simulink library "inp"  (R2021b)
settings: Solver=VariableStepAuto  StartTime=0.0  StopTime=10.0  RelTol=1e-3
undefined symbols (not defined in the file): C_TASK_5MS_S, FALSE, KINP_AcoreReadyToSlp_flg_ovrdflg, KINP_AcoreReadyToSlp_flg_ovrdval, KINP_AllowMovThd_OTA_enum_ovrdflg, KINP_AllowMovThd_OTA_enum_ovrdval, KINP_APSAngleTarget_Deg_ovrdflg, KINP_APSAngleTarget_Deg_ovrdval, KINP_APSDecReq_mps2_ovrdflg, KINP_APSDecReq_mps2_ovrdval, KINP_APSDecReqA_flg_ovrdflg, KINP_APSDecReqA_flg_ovrdval, KINP_APSDFLL_cm_ovrdflg, KINP_APSDFLL_cm_ovrdval, KINP_APSDFLR_cm_ovrdflg, KINP_APSDFLR_cm_ovrdval, KINP_APSDRLL_cm_ovrdflg, KINP_APSDRLL_cm_ovrdval, KINP_APSDRLR_cm_ovrdflg, KINP_APSDRLR_cm_ovrdval, KINP_APSExitCondition_enum_ovrdflg, KINP_APSExitCondition_enum_ovrdval, KINP_APSHWVer_enum_ovrdflg, KINP_APSHWVer_enum_ovrdval, KINP_APSProgressPCT_pct_ovrdflg, KINP_APSProgressPCT_pct_ovrdval, KINP_APSReq_enum_ovrdflg, KINP_APSReq_enum_ovrdval, KINP_APSRQDisplay_enum_ovrdflg, KINP_APSRQDisplay_enum_ovrdval, KINP_APSRqEPASCtrl_flg_ovrdflg, KINP_APSRqEPASCtrl_flg_ovrdval, KINP_APSShiftPosnReq_enum_ovrdval, KINP_APSShiftPosnReq_enum_ovrflg, KINP_APSSpeedCMD_kph_ovrdval, KINP_APSSpeedCMD_kph_ovrflg, KINP_APSStaSystem_enum_ovrdflg, KINP_APSStaSystem_enum_ovrdval, KINP_APSSWVer_enum_ovrdflg, KINP_APSSWVer_enum_ovrdval, KINP_APSVMCReqA_flg_ovrdval, KINP_APSVMCReqA_flg_ovrflg, KINP_APSVRqEPASCtrl_flg_ovrdflg, KINP_APSVRqEPASCtrl_flg_ovrdval, KINP_AuxBattVolmV_mV_ovrdflg, KINP_AuxBattVolmV_mV_ovrdval, KINP_CAASSta_enum_ovrdflg, KINP_CAASSta_enum_ovrdval, KINP_CAASVMCReqA_flg_ovrdval, KINP_CAASVMCReqA_flg_ovrflg, KINP_Chime_enum_ovrdflg, KINP_Chime_enum_ovrdval, KINP_ClearDTCcmd_flg_ovrdflg, KINP_ClearDTCcmd_flg_ovrdval, KINP_EvccAplusPwrUpReq_flg_ovrdflg, KINP_EvccAplusPwrUpReq_flg_ovrdval, KINP_LFID_raw_ovrdval, KINP_LFID_raw_ovrflg, KINP_LRID_raw_ovrdval, KINP_MemOffsetAccX_raw16_ovrdflg ... (+118)
libraries: FVT_lib x942, hcu_lib x1
(part 2 of 31)

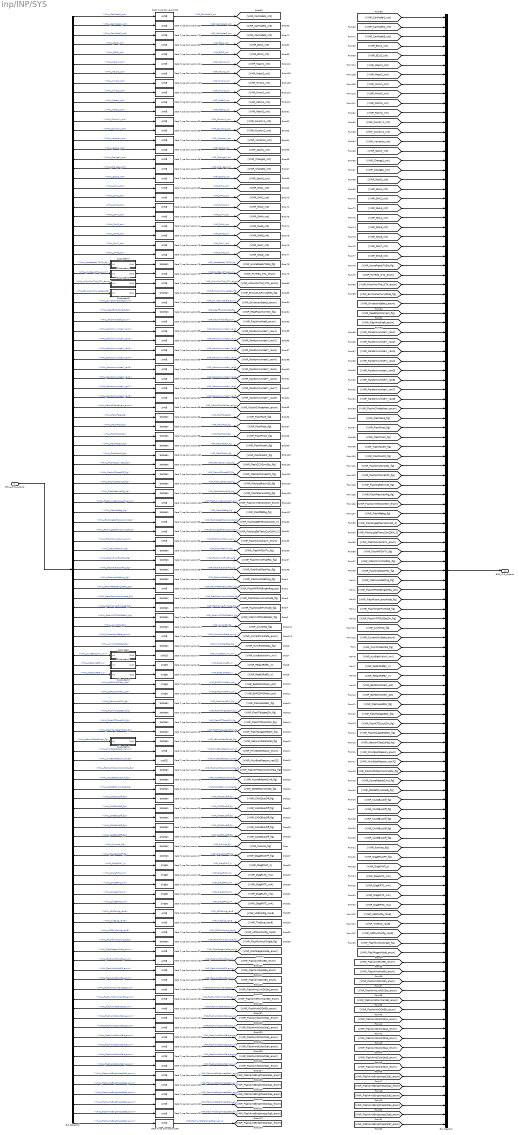
== system inp/INP/SYS ==
  BHAL_SYS_outputs : Inport  OutDataTypeStr=Bus: BHAL_SYS_outputs
  Bus Creator1 : BusCreator  Inputs=117
  Bus Selector1 : BusSelector  OutputSignals=VHAL_CarMode1_cnt,VHAL_CarModel2_cnt,VHAL_CarModel3_cnt,VHAL_ECU1_cnt,VHAL_ECU2_cnt,VHAL_Major1_cnt,VHAL_Major2_cnt,VHAL_Minor1_cnt,VHAL_Minor2_cnt,VHAL_Patch1_cnt,VHAL_Patch2_cnt,VHAL_Country1_cnt,VHAL_Country2_cnt,VHAL_Variation_cnt,VHAL_Dash1_cnt,VHAL_Change1_cnt,VHAL_Change2_cnt,VHAL_Dash2_cnt,VHAL_SHA1_cnt,VHAL_SHA2_cnt,VHAL_SHA3_cnt,VHAL_SHA4_cnt,VHAL_SHA5_cnt,VHAL_SHA6_cnt,VHAL_SHA7_cnt,VHAL_SHA8_cnt,VHAL_AcoreReadyToSlp_flg,VHAL_PwrReq_OTA_enum,VHAL_AllowMovThd_OTA_enum,VHAL_EvccAplusPwrUpReq_flg,VHAL_DrivetrainSelect_enum,VHAL_ReadFlashCorrect_flg,VHAL_FlashAntitheft_enum,VHAL_RandomnumberY_raw1,VHAL_RandomnumberY_raw2,VHAL_RandomnumberY_raw3,VHAL_RandomnumberY_raw4,VHAL_RandomnumberY_raw5,VHAL_RandomnumberY_raw6,VHAL_RandomnumberY_raw7,VHAL_RandomnumberY_raw8,VHAL_FlashACModeMem_enum,VHAL_FlashFace_flg,VHAL_FlashFoot_flg,VHAL_FlashFrost_flg,VHAL_FlashFaceM_flg,VHAL_FlashFootM_flg,VHAL_FlashCCUSyncSts_flg,VHAL_FlashACForceOFF_flg,VHAL_FlashsigRecircSt_flg,VHAL_FlashRecAutoFlg_flg,VHAL_FlashAirIntenZone1M_enum,VHAL_Flashfdefog_flg,VHAL_FlashsigSetTempZon1St_C,VHAL_FlashsigSetTempZon2StM_C,VHAL_FlashCountAlarm_enum,VHAL_FlashMFSWTri_flg,VHAL_FlashMirrorFlodPos_flg,VHAL_FlashFuelDoorPos_flg,VHAL_FlashLockSetting_flg,VHAL_FlashMFRDNBrightReq_pct,VHAL_FlashRoomLampMode_flg,VHAL_FlashWiperFixMode_flg,VHAL_FlashIVIPTGUSStaSW_flg,VHAL_AnyNMID_flg,VHAL_CurrentNmState_enum,VHAL_NvmProtectSta_flg,VHAL_AuxBattVolmV_mV,VHAL_Pedal1Ref5V_V,VHAL_Pedal2Ref5V_V,VHAL_EAPS1MINMem_pct,VHAL_EAPS2MINMem_pct,VHAL_FlashHoodSW_flg,VHAL_FlashTailgateSW_flg,VHAL_FlashCTDLockSW_flg,VHAL_FlashTailgateHDSW_flg,VHAL_NetworkReqCalled_flg,VHAL_PmicBootReason_enum,VHAL_WisrBootReason_raw32,VHAL_FlashAPMDoorControlSta_flg,VHAL_AcoreRebootCmd_flg,VHAL_DIDGetDynoMode_flg,VHAL_CAN1BusOff_flg,VHAL_CAN2BusOff_flg,VHAL_CAN3BusOff_flg,VHAL_CAN4BusOff_flg,VHAL_CAN5BusOff_flg,VHAL_funAuto_flg,VHAL_DiagDRLOFF_flg,VHAL_DiagFMHT_s,VHAL_DiagFLTC_mA,VHAL_DiagFRTC_mA,VHAL_DiagRLTC_mA,VHAL_DiagRRTC_mA,VHAL_USSConfig_raw8,VHAL_TireSize_raw8,VHAL_APSFunConfig_raw8,VHAL_FlashfUnlockSingle_flg,VHAL_FlashRegenMode_enum,VHAL_FlashAmbFunEN_enum,VHAL_FlashAmbWelEN_enum,VHAL_FlashAmbDimEN_enum,VHAL_FlashAmbLinkDriSta_enum,VHAL_FlashAmbPwrWarnEN_enum,VHAL_FlashAmbODAEN_enum,VHAL_FlashAmbColorSta1_enum,VHAL_FlashAmbColorSta2_enum,VHAL_FlashAmbColorSta3_enum,VHAL_FlashAmbColorSta4_enum,VHAL_FlashAmbColorSta5_enum,VHAL_FlashAmbColorSta7_enum,VHAL_FlashAmbBrightnessSta1_enum,VHAL_FlashAmbBrightnessSta2_enum,VHAL_FlashAmbBrightnessSta3_enum,VHAL_FlashAmbBrightnessSta4_enum,VHAL_FlashAmbBrightnessSta5_enum,VHAL_FlashAmbBrightnessSta7_enum
  Data Type Conversion{,1,3..6,12..16,19..27,36,54,57..58,78,81,89,96..103,105,107,112} (38 alike) : DataTypeConversion  OutDataTypeStr=boolean
  Data Type Conversion{8..11,28..32} (9 alike) : DataTypeConversion  OutDataTypeStr=single
  Data Type Conversion{2,17,33..35,37,53,55..56,59..77,79..80,82..88,90..95,104,106,108..111,113,192..209} (68 alike) : DataTypeConversion  OutDataTypeStr=uint8
  Data Type Conversion18 : DataTypeConversion  OutDataTypeStr=uint32
  Data Type Conversion7 : DataTypeConversion  OutDataTypeStr=uint16
  Subsystem : Subsystem
  Subsystem1 : Subsystem
  Subsystem2 : Subsystem
  Subsystem3 : Subsystem
  Subsystem4 : Subsystem
  Subsystem5 : Subsystem
  Subsystem6 : Subsystem
  Subsystem7 : Subsystem
  BINP_SYS_outputs : Outport  OutDataTypeStr=Bus: BINP_SYS_outputs
  wires:
  [VINP_Country2_cnt] -> Bus Creator1/13
  [VINP_FlashAirIntenZone1M_enum] -> Bus Creator1/52
  [VINP_FlashFrost_flg] -> Bus Creator1/45
  Bus Selector1/43 -> Data Type Conversion96/1  "<VHAL_FlashFace_flg>"
  [VINP_FlashCCUSyncSts_flg] -> Bus Creator1/48
  [VINP_EvccAplusPwrUpReq_flg] -> Bus Creator1/30
  Data Type Conversion110/1 -> [VINP_Minor2_cnt]  "VINP_Minor2_cnt"
  Bus Selector1/53 -> Data Type Conversion107/1  "<VHAL_Flashfdefog_flg>"
  [VINP_FlashRecAutoFlg_flg] -> Bus Creator1/51
  Bus Selector1/16 -> Data Type Conversion66/1  "<VHAL_Change1_cnt>"
  [VINP_RandomnumberY_raw1] -> Bus Creator1/34
  Data Type Conversion97/1 -> [VINP_FlashFoot_flg]  "VINP_FlashFoot_flg"
  Bus Selector1/44 -> Data Type Conversion97/1  "<VHAL_FlashFoot_flg>"
  [VINP_FlashFoot_flg] -> Bus Creator1/44
  [VINP_FlashFootM_flg] -> Bus Creator1/47
  Data Type Conversion72/1 -> [VINP_SHA3_cnt]  "VINP_SHA3_cnt"
  [VINP_FlashsigRecircSt_flg] -> Bus Creator1/50
  Data Type Conversion60/1 -> [VINP_CarModel2_cnt]  "VINP_CarModel2_cnt"
  Data Type Conversion100/1 -> [VINP_FlashFootM_flg]  "VINP_FlashFootM_flg"
  Bus Selector1/3 -> Data Type Conversion71/1  "<VHAL_CarModel3_cnt>"
  Data Type Conversion104/1 -> [VINP_Major1_cnt]  "VINP_Major1_cnt"
  [VINP_FlashFaceM_flg] -> Bus Creator1/46
  [VINP_Dash1_cnt] -> Bus Creator1/15
  Bus Selector1/45 -> Data Type Conversion98/1  "<VHAL_FlashFrost_flg>"
  [VINP_FlashACModeMem_enum] -> Bus Creator1/42
  Data Type Conversion108/1 -> [VINP_Major2_cnt]  "VINP_Major2_cnt"
  [VINP_FlashFace_flg] -> Bus Creator1/43
  Bus Selector1/8 -> Data Type Conversion109/1  "<VHAL_Minor1_cnt>"
  [VINP_CarModel1_cnt] -> Bus Creator1/1
  Data Type Conversion82/1 -> [VINP_ECU1_cnt]  "VINP_ECU1_cnt"
  Bus Selector1/47 -> Data Type Conversion100/1  "<VHAL_FlashFootM_flg>"
  Data Type Conversion73/1 -> [VINP_SHA4_cnt]  "VINP_SHA4_cnt"
  Bus Selector1/34 -> Data Type Conversion85/1  "<VHAL_RandomnumberY_raw1>"
  Data Type Conversion84/1 -> [VINP_DrivetrainSelect_enum]  "VINP_DrivetrainSelect_enum"
  Bus Selector1/30 -> Subsystem6/1(In1)  "<VHAL_EvccAplusPwrUpReq_flg>"
  Data Type Conversion101/1 -> [VINP_FlashCCUSyncSts_flg]  "VINP_FlashCCUSyncSts_flg"
  [VINP_DrivetrainSelect_enum] -> Bus Creator1/31
  Data Type Conversion80/1 -> [VINP_AllowMovThd_OTA_enum]  "VINP_AllowMovThd_OTA_enum"
  Bus Selector1/49 -> Data Type Conversion102/1  "<VHAL_FlashACForceOFF_flg>"
  Bus Selector1/38 -> Data Type Conversion90/1  "<VHAL_RandomnumberY_raw5>"
  Bus Selector1/10 -> Data Type Conversion111/1  "<VHAL_Patch1_cnt>"
  Data Type Conversion88/1 -> [VINP_RandomnumberY_raw4]  "VINP_RandomnumberY_raw4"
  [VINP_Flashfdefog_flg] -> Bus Creator1/53
  Bus Selector1/42 -> Data Type Conversion95/1  "<VHAL_FlashACModeMem_enum>"
  Bus Selector1/37 -> Data Type Conversion88/1  "<VHAL_RandomnumberY_raw4>"
  Bus Selector1/36 -> Data Type Conversion87/1  "<VHAL_RandomnumberY_raw3>"
  Bus Selector1/48 -> Data Type Conversion101/1  "<VHAL_FlashCCUSyncSts_flg>"
  Data Type Conversion102/1 -> [VINP_FlashACForceOFF_flg]  "VINP_FlashACForceOFF_flg"
  [VINP_Change2_cnt] -> Bus Creator1/17
  Bus Selector1/29 -> Subsystem5/1(In1)  "<VHAL_AllowMovThd_OTA_enum>"
  Data Type Conversion63/1 -> [VINP_Country2_cnt]  "VINP_Country2_cnt"
  Data Type Conversion107/1 -> [VINP_Flashfdefog_flg]  "VINP_Flashfdefog_flg"
  Data Type Conversion96/1 -> [VINP_FlashFace_flg]  "VINP_FlashFace_flg"
  [VINP_RandomnumberY_raw2] -> Bus Creator1/35
  [VINP_RandomnumberY_raw6] -> Bus Creator1/39
  [VINP_RandomnumberY_raw4] -> Bus Creator1/37
  [VINP_ECU1_cnt] -> Bus Creator1/4
  Bus Selector1/2 -> Data Type Conversion60/1  "<VHAL_CarModel2_cnt>"
  Data Type Conversion105/1 -> [VINP_FlashRecAutoFlg_flg]  "VINP_FlashRecAutoFlg_flg"
  Data Type Conversion103/1 -> [VINP_FlashsigRecircSt_flg]  "VINP_FlashsigRecircSt_flg"
  Bus Selector1/22 -> Data Type Conversion73/1  "<VHAL_SHA4_cnt>"
  Bus Selector1/46 -> Data Type Conversion99/1  "<VHAL_FlashFaceM_flg>"
  Bus Selector1/50 -> Data Type Conversion103/1  "<VHAL_FlashsigRecircSt_flg>"
  Data Type Conversion98/1 -> [VINP_FlashFrost_flg]  "VINP_FlashFrost_flg"
  [VINP_RandomnumberY_raw5] -> Bus Creator1/38
  [VINP_SHA3_cnt] -> Bus Creator1/21
  Bus Selector1/40 -> Data Type Conversion92/1  "<VHAL_RandomnumberY_raw7>"
  Data Type Conversion86/1 -> [VINP_RandomnumberY_raw2]  "VINP_RandomnumberY_raw2"
  Data Type Conversion111/1 -> [VINP_Patch1_cnt]  "VINP_Patch1_cnt"
  Bus Selector1/35 -> Data Type Conversion86/1  "<VHAL_RandomnumberY_raw2>"
  [VINP_SHA6_cnt] -> Bus Creator1/24
  [VINP_Major1_cnt] -> Bus Creator1/6
  [VINP_RandomnumberY_raw7] -> Bus Creator1/40
  [VINP_RandomnumberY_raw8] -> Bus Creator1/41
  Bus Selector1/15 -> Data Type Conversion65/1  "<VHAL_Dash1_cnt>"
  Data Type Conversion92/1 -> [VINP_RandomnumberY_raw7]  "VINP_RandomnumberY_raw7"
  Data Type Conversion99/1 -> [VINP_FlashFaceM_flg]  "VINP_FlashFaceM_flg"
  Data Type Conversion85/1 -> [VINP_RandomnumberY_raw1]  "VINP_RandomnumberY_raw1"
  Bus Selector1/52 -> Data Type Conversion106/1  "<VHAL_FlashAirIntenZone1M_enum>"
  Data Type Conversion90/1 -> [VINP_RandomnumberY_raw5]  "VINP_RandomnumberY_raw5"
  Data Type Conversion91/1 -> [VINP_RandomnumberY_raw6]  "VINP_RandomnumberY_raw6"
  Data Type Conversion65/1 -> [VINP_Dash1_cnt]  "VINP_Dash1_cnt"
  [VINP_FlashAntitheft_enum] -> Bus Creator1/33
  Data Type Conversion87/1 -> [VINP_RandomnumberY_raw3]  "VINP_RandomnumberY_raw3"
  Bus Selector1/39 -> Data Type Conversion91/1  "<VHAL_RandomnumberY_raw6>"
  [VINP_Dash2_cnt] -> Bus Creator1/18
  Bus Selector1/19 -> Data Type Conversion69/1  "<VHAL_SHA1_cnt>"
  Bus Selector1/41 -> Data Type Conversion94/1  "<VHAL_RandomnumberY_raw8>"
  Data Type Conversion71/1 -> [VINP_CarModel3_cnt]  "VINP_CarModel3_cnt"
  [VINP_SHA4_cnt] -> Bus Creator1/22
  Data Type Conversion76/1 -> [VINP_SHA7_cnt]  "VINP_SHA7_cnt"
  [VINP_AllowMovThd_OTA_enum] -> Bus Creator1/29
  [VINP_ReadFlashCorrect_flg] -> Bus Creator1/32
  Data Type Conversion78/1 -> [VINP_AcoreReadyToSlp_flg]  "VINP_AcoreReadyToSlp_flg"
  Data Type Conversion94/1 -> [VINP_RandomnumberY_raw8]  "VINP_RandomnumberY_raw8"
  Data Type Conversion67/1 -> [VINP_Change2_cnt]  "VINP_Change2_cnt"
  [VINP_CarModel3_cnt] -> Bus Creator1/3
  [VINP_Variation_cnt] -> Bus Creator1/14
  [VINP_SHA2_cnt] -> Bus Creator1/20
  [VINP_FlashACForceOFF_flg] -> Bus Creator1/49
  Bus Selector1/12 -> Data Type Conversion62/1  "<VHAL_Country1_cnt>"
  Bus Selector1/51 -> Data Type Conversion105/1  "<VHAL_FlashRecAutoFlg_flg>"
  Data Type Conversion69/1 -> [VINP_SHA1_cnt]  "VINP_SHA1_cnt"
  [VINP_AcoreReadyToSlp_flg] -> Bus Creator1/27
  [VINP_PwrReq_OTA_enum] -> Bus Creator1/28
  Subsystem4/1(Out1) -> Data Type Conversion79/1
  [VINP_SHA5_cnt] -> Bus Creator1/23
  [VINP_Patch2_cnt] -> Bus Creator1/11
  [VINP_Patch1_cnt] -> Bus Creator1/10
  Data Type Conversion68/1 -> [VINP_Dash2_cnt]  "VINP_Dash2_cnt"
  Subsystem6/1(Out1) -> Data Type Conversion89/1
  Bus Selector1/33 -> Data Type Conversion83/1  "<VHAL_FlashAntitheft_enum>"
  [VINP_Minor2_cnt] -> Bus Creator1/9
  [VINP_SHA7_cnt] -> Bus Creator1/25
  [VINP_Minor1_cnt] -> Bus Creator1/8
  Data Type Conversion95/1 -> [VINP_FlashACModeMem_enum]  "VINP_FlashACModeMem_enum"
  [VINP_CarModel2_cnt] -> Bus Creator1/2
  Data Type Conversion77/1 -> [VINP_SHA8_cnt]  "VINP_SHA8_cnt"
  Data Type Conversion106/1 -> [VINP_FlashAirIntenZone1M_enum]  "VINP_FlashAirIntenZone1M_enum"
  Data Type Conversion66/1 -> [VINP_Change1_cnt]  "VINP_Change1_cnt"
  [VINP_SHA1_cnt] -> Bus Creator1/19
  Data Type Conversion81/1 -> [VINP_ReadFlashCorrect_flg]  "VINP_ReadFlashCorrect_flg"
  [VINP_Country1_cnt] -> Bus Creator1/12
  Bus Selector1/17 -> Data Type Conversion67/1  "<VHAL_Change2_cnt>"
  Data Type Conversion83/1 -> [VINP_FlashAntitheft_enum]  "VINP_FlashAntitheft_enum"
  Data Type Conversion75/1 -> [VINP_SHA6_cnt]  "VINP_SHA6_cnt"
  Data Type Conversion74/1 -> [VINP_SHA5_cnt]  "VINP_SHA5_cnt"
  Data Type Conversion93/1 -> [VINP_ECU2_cnt]  "VINP_ECU2_cnt"
  [VINP_RandomnumberY_raw3] -> Bus Creator1/36
  Data Type Conversion70/1 -> [VINP_SHA2_cnt]  "VINP_SHA2_cnt"
  Bus Selector1/21 -> Data Type Conversion72/1  "<VHAL_SHA3_cnt>"
  Data Type Conversion62/1 -> [VINP_Country1_cnt]  "VINP_Country1_cnt"
  [VINP_ECU2_cnt] -> Bus Creator1/5
  Bus Selector1/31 -> Data Type Conversion84/1  "<VHAL_DrivetrainSelect_enum>"
  Data Type Conversion64/1 -> [VINP_Variation_cnt]  "VINP_Variation_cnt"
  Data Type Conversion61/1 -> [VINP_Patch2_cnt]  "VINP_Patch2_cnt"
  Bus Selector1/18 -> Data Type Conversion68/1  "<VHAL_Dash2_cnt>"
  Bus Selector1/28 -> Subsystem4/1(In1)  "<VHAL_PwrReq_OTA_enum>"
  Bus Selector1/24 -> Data Type Conversion75/1  "<VHAL_SHA6_cnt>"
  Bus Selector1/27 -> Subsystem7/1(In1)  "<VHAL_AcoreReadyToSlp_flg>"
  [VINP_SHA8_cnt] -> Bus Creator1/26
  Bus Selector1/20 -> Data Type Conversion70/1  "<VHAL_SHA2_cnt>"
  Subsystem5/1(Out1) -> Data Type Conversion80/1
  Bus Selector1/25 -> Data Type Conversion76/1  "<VHAL_SHA7_cnt>"
  [VINP_Major2_cnt] -> Bus Creator1/7
  Bus Selector1/32 -> Data Type Conversion81/1  "<VHAL_ReadFlashCorrect_flg>"
  Data Type Conversion59/1 -> [VINP_CarModel1_cnt]  "VINP_CarModel1_cnt"
  Bus Selector1/23 -> Data Type Conversion74/1  "<VHAL_SHA5_cnt>"
  Bus Selector1/14 -> Data Type Conversion64/1  "<VHAL_Variation_cnt>"
  [VINP_Change1_cnt] -> Bus Creator1/16
  Subsystem7/1(Out1) -> Data Type Conversion78/1
  Bus Selector1/13 -> Data Type Conversion63/1  "<VHAL_Country2_cnt>"
  Bus Selector1/4 -> Data Type Conversion82/1  "<VHAL_ECU1_cnt>"
  Data Type Conversion79/1 -> [VINP_PwrReq_OTA_enum]  "VINP_PwrReq_OTA_enum"
  Bus Selector1/7 -> Data Type Conversion108/1  "<VHAL_Major2_cnt>"
  Bus Selector1/9 -> Data Type Conversion110/1  "<VHAL_Minor2_cnt>"
  Bus Selector1/5 -> Data Type Conversion93/1  "<VHAL_ECU2_cnt>"
  Data Type Conversion89/1 -> [VINP_EvccAplusPwrUpReq_flg]  "VINP_EvccAplusPwrUpReq_flg"
  Bus Selector1/1 -> Data Type Conversion59/1  "<VHAL_CarMode1_cnt>"
  Bus Selector1/6 -> Data Type Conversion104/1  "<VHAL_Major1_cnt>"
  Data Type Conversion109/1 -> [VINP_Minor1_cnt]  "VINP_Minor1_cnt"
  BHAL_SYS_outputs/1 -> Bus Selector1/1
  Bus Creator1/1 -> BINP_SYS_outputs/1
  Bus Selector1/11 -> Data Type Conversion61/1  "<VHAL_Patch2_cnt>"
  Bus Selector1/26 -> Data Type Conversion77/1  "<VHAL_SHA8_cnt>"
  Data Type Conversion112/1 -> [VINP_AnyNMID_flg]  "VINP_AnyNMID_flg"
  Data Type Conversion113/1 -> [VINP_CurrentNmState_enum]  "VINP_CurrentNmState_enum"
  Bus Selector1/65 -> Data Type Conversion112/1  "<VHAL_AnyNMID_flg>"
  Bus Selector1/66 -> Data Type Conversion113/1  "<VHAL_CurrentNmState_enum>"
  Data Type Conversion56/1 -> [VINP_FlashCountAlarm_enum]  "VINP_FlashCountAlarm_enum"
  Data Type Conversion4/1 -> [VINP_FlashWiperFixMode_flg]  "VINP_FlashWiperFixMode_flg"
  Data Type Conversion3/1 -> [VINP_FlashRoomLampMode_flg]  "VINP_FlashRoomLampMode_flg"
  Data Type Conversion57/1 -> [VINP_FlashMirrorFlodPos_flg]  "VINP_FlashMirrorFlodPos_flg"
  Data Type Conversion55/1 -> [VINP_FlashsigSetTempZon2StM_C]  "VINP_FlashsigSetTempZon2StM_C"
  Data Type Conversion54/1 -> [VINP_FlashMFSWTri_flg]  "VINP_FlashMFSWTri_flg"
  Data Type Conversion58/1 -> [VINP_FlashFuelDoorPos_flg]  "VINP_FlashFuelDoorPos_flg"
  Data Type Conversion53/1 -> [VINP_FlashsigSetTempZon1St_C]  "VINP_FlashsigSetTempZon1St_C"
  Data Type Conversion5/1 -> [VINP_FlashIVIPTGUSStaSW_flg]  "VINP_FlashIVIPTGUSStaSW_flg"
  Data Type Conversion2/1 -> [VINP_FlashMFRDNBrightReq_pct]  "VINP_FlashMFRDNBrightReq_pct"
  Data Type Conversion1/1 -> [VINP_FlashLockSetting_flg]  "VINP_FlashLockSetting_flg"
  Bus Selector1/54 -> Data Type Conversion53/1  "<VHAL_FlashsigSetTempZon1St_C>"
  Bus Selector1/55 -> Data Type Conversion55/1  "<VHAL_FlashsigSetTempZon2StM_C>"
  Bus Selector1/56 -> Data Type Conversion56/1  "<VHAL_FlashCountAlarm_enum>"
  Bus Selector1/57 -> Data Type Conversion54/1  "<VHAL_FlashMFSWTri_flg>"
  Bus Selector1/58 -> Data Type Conversion57/1  "<VHAL_FlashMirrorFlodPos_flg>"
  Bus Selector1/59 -> Data Type Conversion58/1  "<VHAL_FlashFuelDoorPos_flg>"
  Bus Selector1/60 -> Data Type Conversion1/1  "<VHAL_FlashLockSetting_flg>"
  Bus Selector1/61 -> Data Type Conversion2/1  "<VHAL_FlashMFRDNBrightReq_pct>"
  Bus Selector1/62 -> Data Type Conversion3/1  "<VHAL_FlashRoomLampMode_flg>"
  Bus Selector1/63 -> Data Type Conversion4/1  "<VHAL_FlashWiperFixMode_flg>"
  Bus Selector1/64 -> Data Type Conversion5/1  "<VHAL_FlashIVIPTGUSStaSW_flg>"
  [VINP_FlashsigSetTempZon1St_C] -> Bus Creator1/54
  [VINP_FlashsigSetTempZon2StM_C] -> Bus Creator1/55
  [VINP_FlashCountAlarm_enum] -> Bus Creator1/56
  [VINP_FlashMFSWTri_flg] -> Bus Creator1/57
  [VINP_FlashMirrorFlodPos_flg] -> Bus Creator1/58
  [VINP_FlashFuelDoorPos_flg] -> Bus Creator1/59
  [VINP_FlashLockSetting_flg] -> Bus Creator1/60
  [VINP_FlashMFRDNBrightReq_pct] -> Bus Creator1/61
  [VINP_FlashRoomLampMode_flg] -> Bus Creator1/62
  [VINP_FlashWiperFixMode_flg] -> Bus Creator1/63
  [VINP_FlashIVIPTGUSStaSW_flg] -> Bus Creator1/64
  [VINP_AnyNMID_flg] -> Bus Creator1/65
  [VINP_CurrentNmState_enum] -> Bus Creator1/66
  Bus Selector1/67 -> Data Type Conversion6/1  "<VHAL_NvmProtectSta_flg>"
  Data Type Conversion6/1 -> [VINP_NvmProtectSta_flg]  "VINP_NvmProtectSta_flg"
  [VINP_NvmProtectSta_flg] -> Bus Creator1/67
  Bus Selector1/68 -> Subsystem/1(In1)  "<VHAL_AuxBattVolmV_mV>"
  Bus Selector1/69 -> Subsystem2/1(In1)  "<VHAL_Pedal1Ref5V_V>"
  Bus Selector1/70 -> Subsystem3/1(In1)  "<VHAL_Pedal2Ref5V_V>"
  Bus Selector1/71 -> Data Type Conversion10/1  "<VHAL_EAPS1MINMem_pct>"
  Bus Selector1/72 -> Data Type Conversion11/1  "<VHAL_EAPS2MINMem_pct>"
  Data Type Conversion7/1 -> [VINP_AuxBattVolmV_mV]  "VINP_AuxBattVolmV_mV"
  Data Type Conversion8/1 -> [VINP_Pedal1Ref5V_V]  "VINP_Pedal1Ref5V_V"
  Data Type Conversion9/1 -> [VINP_Pedal2Ref5V_V]  "VINP_Pedal2Ref5V_V"
  Data Type Conversion10/1 -> [VINP_EAPS1MINMem_pct]  "VINP_EAPS1MINMem_pct"
  Data Type Conversion11/1 -> [VINP_EAPS2MINMem_pct]  "VINP_EAPS2MINMem_pct"
  [VINP_AuxBattVolmV_mV] -> Bus Creator1/68
  [VINP_Pedal1Ref5V_V] -> Bus Creator1/69
  [VINP_Pedal2Ref5V_V] -> Bus Creator1/70
  [VINP_EAPS1MINMem_pct] -> Bus Creator1/71
  [VINP_EAPS2MINMem_pct] -> Bus Creator1/72
  Bus Selector1/73 -> Data Type Conversion12/1  "<VHAL_FlashHoodSW_flg>"
  Bus Selector1/74 -> Data Type Conversion13/1  "<VHAL_FlashTailgateSW_flg>"
  Bus Selector1/75 -> Data Type Conversion14/1  "<VHAL_FlashCTDLockSW_flg>"
  Bus Selector1/76 -> Data Type Conversion15/1  "<VHAL_FlashTailgateHDSW_flg>"
  Data Type Conversion12/1 -> [VINP_FlashHoodSW_flg]  "VINP_FlashHoodSW_flg"
  Data Type Conversion13/1 -> [VINP_FlashTailgateSW_flg]  "VINP_FlashTailgateSW_flg"
  Data Type Conversion14/1 -> [VINP_FlashCTDLockSW_flg]  "VINP_FlashCTDLockSW_flg"
  Data Type Conversion15/1 -> [VINP_FlashTailgateHDSW_flg]  "VINP_FlashTailgateHDSW_flg"
  [VINP_FlashHoodSW_flg] -> Bus Creator1/73
  [VINP_FlashTailgateSW_flg] -> Bus Creator1/74
  [VINP_FlashCTDLockSW_flg] -> Bus Creator1/75
  [VINP_FlashTailgateHDSW_flg] -> Bus Creator1/76
  Subsystem/1(Out1) -> Data Type Conversion7/1
  Bus Selector1/77 -> Subsystem1/1(In1)  "<VHAL_NetworkReqCalled_flg>"
  Data Type Conversion16/1 -> [VINP_NetworkReqCalled_flg]  "VINP_NetworkReqCalled_flg"
  Subsystem1/1(Out1) -> Data Type Conversion16/1
  [VINP_NetworkReqCalled_flg] -> Bus Creator1/77
  Bus Selector1/78 -> Data Type Conversion17/1  "<VHAL_PmicBootReason_enum>"
  Bus Selector1/79 -> Data Type Conversion18/1  "<VHAL_WisrBootReason_raw32>"
  Bus Selector1/80 -> Data Type Conversion19/1  "<VHAL_FlashAPMDoorControlSta_flg>"
  Data Type Conversion17/1 -> [VINP_PmicBootReason_enum]  "VINP_PmicBootReason_enum"
  Data Type Conversion18/1 -> [VINP_WisrBootReason_raw32]  "VINP_WisrBootReason_raw32"
  Data Type Conversion19/1 -> [VINP_FlashAPMDoorControlSta_flg]  "VINP_FlashAPMDoorControlSta_flg"
  [VINP_PmicBootReason_enum] -> Bus Creator1/78
  [VINP_WisrBootReason_raw32] -> Bus Creator1/79
  [VINP_FlashAPMDoorControlSta_flg] -> Bus Creator1/80
  Subsystem2/1(Out1) -> Data Type Conversion8/1
  Subsystem3/1(Out1) -> Data Type Conversion9/1
  Bus Selector1/81 -> Data Type Conversion20/1  "<VHAL_AcoreRebootCmd_flg>"
  Data Type Conversion20/1 -> [VINP_AcoreRebootCmd_flg]  "VINP_AcoreRebootCmd_flg"
  [VINP_AcoreRebootCmd_flg] -> Bus Creator1/81
  Bus Selector1/82 -> Data Type Conversion21/1  "<VHAL_DIDGetDynoMode_flg>"
  Data Type Conversion21/1 -> [VINP_DIDGetDynoMode_flg]  "VINP_DIDGetDynoMode_flg"
  [VINP_DIDGetDynoMode_flg] -> Bus Creator1/82
  Bus Selector1/83 -> Data Type Conversion22/1  "<VHAL_CAN1BusOff_flg>"
  Bus Selector1/84 -> Data Type Conversion23/1  "<VHAL_CAN2BusOff_flg>"
  Bus Selector1/85 -> Data Type Conversion24/1  "<VHAL_CAN3BusOff_flg>"
  Bus Selector1/86 -> Data Type Conversion25/1  "<VHAL_CAN4BusOff_flg>"
  Bus Selector1/87 -> Data Type Conversion26/1  "<VHAL_CAN5BusOff_flg>"
  Data Type Conversion22/1 -> [VINP_CAN1BusOff_flg]  "VINP_CAN1BusOff_flg"
  Data Type Conversion23/1 -> [VINP_CAN2BusOff_flg]  "VINP_CAN2BusOff_flg"
  Data Type Conversion24/1 -> [VINP_CAN3BusOff_flg]  "VINP_CAN3BusOff_flg"
  Data Type Conversion25/1 -> [VINP_CAN4BusOff_flg]  "VINP_CAN4BusOff_flg"
  Data Type Conversion26/1 -> [VINP_CAN5BusOff_flg]  "VINP_CAN5BusOff_flg"
  [VINP_CAN1BusOff_flg] -> Bus Creator1/83
  [VINP_CAN2BusOff_flg] -> Bus Creator1/84
  [VINP_CAN3BusOff_flg] -> Bus Creator1/85
  [VINP_CAN4BusOff_flg] -> Bus Creator1/86
  [VINP_CAN5BusOff_flg] -> Bus Creator1/87
  Data Type Conversion31/1 -> [VINP_DiagRLTC_mA]  "VINP_DiagRLTC_mA"
  Data Type Conversion29/1 -> [VINP_DiagFLTC_mA]  "VINP_DiagFLTC_mA"
  Bus Selector1/94 -> Data Type Conversion32/1  "<VHAL_DiagRRTC_mA>"
  Data Type Conversion28/1 -> [VINP_DiagFMHT_s]  "VINP_DiagFMHT_s"
  Data Type Conversion32/1 -> [VINP_DiagRRTC_mA]  "VINP_DiagRRTC_mA"
  Data Type Conversion27/1 -> [VINP_DiagDRLOFF_flg]  "VINP_DiagDRLOFF_flg"
  Data Type Conversion30/1 -> [VINP_DiagFRTC_mA]  "VINP_DiagFRTC_mA"
  Bus Selector1/93 -> Data Type Conversion31/1  "<VHAL_DiagRLTC_mA>"
  Bus Selector1/91 -> Data Type Conversion29/1  "<VHAL_DiagFLTC_mA>"
  Data Type Conversion/1 -> [VINP_funAuto_flg]  "VINP_funAuto_flg"
  Bus Selector1/89 -> Data Type Conversion27/1  "<VHAL_DiagDRLOFF_flg>"
  Bus Selector1/90 -> Data Type Conversion28/1  "<VHAL_DiagFMHT_s>"
  Bus Selector1/92 -> Data Type Conversion30/1  "<VHAL_DiagFRTC_mA>"
  Bus Selector1/88 -> Data Type Conversion/1  "<VHAL_funAuto_flg>"
  [VINP_DiagRRTC_mA] -> Bus Creator1/94
  [VINP_DiagRLTC_mA] -> Bus Creator1/93
  [VINP_DiagFRTC_mA] -> Bus Creator1/92
  [VINP_DiagDRLOFF_flg] -> Bus Creator1/89
  [VINP_DiagFLTC_mA] -> Bus Creator1/91
  [VINP_funAuto_flg] -> Bus Creator1/88
  [VINP_DiagFMHT_s] -> Bus Creator1/90
  Bus Selector1/95 -> Data Type Conversion33/1  "<VHAL_USSConfig_raw8>"
  Bus Selector1/96 -> Data Type Conversion34/1  "<VHAL_TireSize_raw8>"
  Bus Selector1/97 -> Data Type Conversion35/1  "<VHAL_APSFunConfig_raw8>"
  [VINP_USSConfig_raw8] -> Bus Creator1/95
  [VINP_TireSize_raw8] -> Bus Creator1/96
  [VINP_APSFunConfig_raw8] -> Bus Creator1/97
  Data Type Conversion33/1 -> [VINP_USSConfig_raw8]  "VINP_USSConfig_raw8"
  Data Type Conversion34/1 -> [VINP_TireSize_raw8]  "VINP_TireSize_raw8"
  Data Type Conversion35/1 -> [VINP_APSFunConfig_raw8]  "VINP_APSFunConfig_raw8"
  Data Type Conversion36/1 -> [VINP_FlashfUnlockSingle_flg]  "VINP_FlashfUnlockSingle_flg"
  Bus Selector1/98 -> Data Type Conversion36/1  "<VHAL_FlashfUnlockSingle_flg>"
  [VINP_FlashfUnlockSingle_flg] -> Bus Creator1/98
  Bus Selector1/99 -> Data Type Conversion37/1  "<VHAL_FlashRegenMode_enum>"
  Data Type Conversion37/1 -> [VINP_FlashRegenMode_enum]  "VINP_FlashRegenMode_enum"
  [VINP_FlashRegenMode_enum] -> Bus Creator1/99
  Data Type Conversion205/1 -> [VINP_FlashAmbBrightnessSta2_enum]  "VINP_FlashAmbBrightnessSta2_enum"
  Bus Selector1/114 -> Data Type Conversion206/1  "<VHAL_FlashAmbBrightnessSta3_enum>"
  Data Type Conversion208/1 -> [VINP_FlashAmbBrightnessSta5_enum]  "VINP_FlashAmbBrightnessSta5_enum"
  Data Type Conversion198/1 -> [VINP_FlashAmbODAEN_enum]  "VINP_FlashAmbODAEN_enum"
  Bus Selector1/104 -> Data Type Conversion197/1  "<VHAL_FlashAmbPwrWarnEN_enum>"
  Bus Selector1/102 -> Data Type Conversion195/1  "<VHAL_FlashAmbDimEN_enum>"
  Data Type Conversion203/1 -> [VINP_FlashAmbColorSta7_enum]  "VINP_FlashAmbColorSta7_enum"
  Bus Selector1/113 -> Data Type Conversion205/1  "<VHAL_FlashAmbBrightnessSta2_enum>"
  Bus Selector1/100 -> Data Type Conversion193/1  "<VHAL_FlashAmbFunEN_enum>"
  Bus Selector1/108 -> Data Type Conversion200/1  "<VHAL_FlashAmbColorSta3_enum>"
  Data Type Conversion192/1 -> [VINP_FlashAmbColorSta1_enum]  "VINP_FlashAmbColorSta1_enum"
  Data Type Conversion194/1 -> [VINP_FlashAmbWelEN_enum]  "VINP_FlashAmbWelEN_enum"
  Data Type Conversion204/1 -> [VINP_FlashAmbBrightnessSta1_enum]  "VINP_FlashAmbBrightnessSta1_enum"
  Bus Selector1/116 -> Data Type Conversion208/1  "<VHAL_FlashAmbBrightnessSta5_enum>"
  Bus Selector1/117 -> Data Type Conversion209/1  "<VHAL_FlashAmbBrightnessSta7_enum>"
  Bus Selector1/112 -> Data Type Conversion204/1  "<VHAL_FlashAmbBrightnessSta1_enum>"
  Bus Selector1/107 -> Data Type Conversion199/1  "<VHAL_FlashAmbColorSta2_enum>"
  Bus Selector1/110 -> Data Type Conversion202/1  "<VHAL_FlashAmbColorSta5_enum>"
  Bus Selector1/106 -> Data Type Conversion192/1  "<VHAL_FlashAmbColorSta1_enum>"
  Data Type Conversion209/1 -> [VINP_FlashAmbBrightnessSta7_enum]  "VINP_FlashAmbBrightnessSta7_enum"
  Bus Selector1/109 -> Data Type Conversion201/1  "<VHAL_FlashAmbColorSta4_enum>"
  Data Type Conversion196/1 -> [VINP_FlashAmbLinkDriSta_enum]  "VINP_FlashAmbLinkDriSta_enum"
  Data Type Conversion199/1 -> [VINP_FlashAmbColorSta2_enum]  "VINP_FlashAmbColorSta2_enum"
  Bus Selector1/103 -> Data Type Conversion196/1  "<VHAL_FlashAmbLinkDriSta_enum>"
  Bus Selector1/105 -> Data Type Conversion198/1  "<VHAL_FlashAmbODAEN_enum>"
  Data Type Conversion195/1 -> [VINP_FlashAmbDimEN_enum]  "VINP_FlashAmbDimEN_enum"
  Bus Selector1/111 -> Data Type Conversion203/1  "<VHAL_FlashAmbColorSta7_enum>"
  Bus Selector1/101 -> Data Type Conversion194/1  "<VHAL_FlashAmbWelEN_enum>"
  Data Type Conversion201/1 -> [VINP_FlashAmbColorSta4_enum]  "VINP_FlashAmbColorSta4_enum"
  Data Type Conversion207/1 -> [VINP_FlashAmbBrightnessSta4_enum]  "VINP_FlashAmbBrightnessSta4_enum"
  Data Type Conversion197/1 -> [VINP_FlashAmbPwrWarnEN_enum]  "VINP_FlashAmbPwrWarnEN_enum"
  Data Type Conversion206/1 -> [VINP_FlashAmbBrightnessSta3_enum]  "VINP_FlashAmbBrightnessSta3_enum"
  Data Type Conversion200/1 -> [VINP_FlashAmbColorSta3_enum]  "VINP_FlashAmbColorSta3_enum"
  Data Type Conversion202/1 -> [VINP_FlashAmbColorSta5_enum]  "VINP_FlashAmbColorSta5_enum"
  Data Type Conversion193/1 -> [VINP_FlashAmbFunEN_enum]  "VINP_FlashAmbFunEN_enum"
  Bus Selector1/115 -> Data Type Conversion207/1  "<VHAL_FlashAmbBrightnessSta4_enum>"
  [VINP_FlashAmbFunEN_enum] -> Bus Creator1/100
  [VINP_FlashAmbWelEN_enum] -> Bus Creator1/101
  [VINP_FlashAmbDimEN_enum] -> Bus Creator1/102
  [VINP_FlashAmbLinkDriSta_enum] -> Bus Creator1/103
  [VINP_FlashAmbPwrWarnEN_enum] -> Bus Creator1/104
  [VINP_FlashAmbODAEN_enum] -> Bus Creator1/105
  [VINP_FlashAmbColorSta1_enum] -> Bus Creator1/106
  [VINP_FlashAmbColorSta2_enum] -> Bus Creator1/107
  [VINP_FlashAmbColorSta3_enum] -> Bus Creator1/108
  [VINP_FlashAmbColorSta4_enum] -> Bus Creator1/109
  [VINP_FlashAmbColorSta5_enum] -> Bus Creator1/110
  [VINP_FlashAmbColorSta7_enum] -> Bus Creator1/111
  [VINP_FlashAmbBrightnessSta1_enum] -> Bus Creator1/112
  [VINP_FlashAmbBrightnessSta2_enum] -> Bus Creator1/113
  [VINP_FlashAmbBrightnessSta3_enum] -> Bus Creator1/114
  [VINP_FlashAmbBrightnessSta4_enum] -> Bus Creator1/115
  [VINP_FlashAmbBrightnessSta5_enum] -> Bus Creator1/116
  [VINP_FlashAmbBrightnessSta7_enum] -> Bus Creator1/117

== system inp/INP/Subsystem ==
  BHAL_DDM_outputs : Inport
  Bus Creator : BusCreator  Inputs=1
  Bus Selector : BusSelector  OutputSignals=VHAL_ClearDTCcmd_flg
  Data Type Conversion12 : DataTypeConversion  OutDataTypeStr=boolean
  Subsystem13 : Subsystem
  BINP_DDM_outputs : Outport
  wires:
  Bus Selector/1 -> Subsystem13/1(In1)  "<VHAL_ClearDTCcmd_flg>"
  Subsystem13/1(Out1) -> Data Type Conversion12/1
  BHAL_DDM_outputs/1 -> Bus Selector/1
  Data Type Conversion12/1 -> Bus Creator/1  "VINP_ClearDTCcmd_flg"
  Bus Creator/1 -> BINP_DDM_outputs/1

== system inp/INP/TPMS ==
  BHAL_TPMS_outputs : Inport  OutDataTypeStr=Bus: BHAL_TPMS_outputs
  Bus Creator : BusCreator  Inputs=50  OutDataTypeStr=Bus: BINP_TPMS_outputs  NonVirtualBus=on
  Bus Selector : BusSelector  OutputSignals=VHAL_TPMSDataIn_flg,VHAL_TPMSID_raw,VHAL_TPMSPressure_raw,VHAL_TPMSTemp_raw,VHAL_TPMSSta_enum,VHAL_TPMSPressureMi_raw,VHAL_TPMSCRC_crc,VHAL_TPMSCRCCalc_crc,VHAL_TPMSFAT_flg,VHAL_TPMSBattLow_flg,VHAL_TPMSStorge_flg,VHAL_LFID_raw,VHAL_RFID_raw,VHAL_LRID_raw,VHAL_RRID_raw,VHAL_ChkStorge_flg,VHAL_ChkLFID_raw,VHAL_ChkRFID_raw,VHAL_ChkLRID_raw,VHAL_ChkRRID_raw,VHAL_FlashLFSensorFail_flg,VHAL_FlashRFSensorFail_flg,VHAL_FlashLRSensorFail_flg,VHAL_FlashRRSensorFail_flg,VHAL_FlashLFWheelPSW_raw8,VHAL_FlashRFWheelPSW_raw8,VHAL_FlashLRWheelPSW_raw8,VHAL_FlashRRWheelPSW_raw8,VHAL_FlashLFPindi_enum,VHAL_FlashRFPindi_enum,VHAL_FlashLRPindi_enum,VHAL_FlashRRPindi_enum,VHAL_FlashLFP20_raw8,VHAL_FlashRFP20_raw8,VHAL_FlashLRP20_raw8,VHAL_FlashRRP20_raw8,VHAL_FlashLFWheelPress_raw8,VHAL_FlashRFWheelPress_raw8,VHAL_FlashLRWheelPress_raw8,VHAL_FlashRRWheelPress_raw8,VHAL_FlashLFWheelTemp_C,VHAL_FlashRFWheelTemp_C,VHAL_FlashLRWheelTemp_C,VHAL_FlashRRWheelTemp_C,VHAL_FlashunlearnSfali_flg,VHAL_S1ID_raw,VHAL_S2ID_raw,VHAL_S3ID_raw,VHAL_S4ID_raw,VHAL_Prepresstemptrust_flg
  Data Type Conversion{,8..10,15,26,45..48,55} (11 alike) : DataTypeConversion  OutDataTypeStr=boolean
  Data Type Conversion{1,11..14,16..19,22..25} (13 alike) : DataTypeConversion  OutDataTypeStr=uint32
  Data Type Conversion{2..7,20..21,32,34..35,37..44,49..54,56} (26 alike) : DataTypeConversion  OutDataTypeStr=uint8
  Subsystem : Subsystem
  Subsystem1 : Subsystem
  Subsystem10 : Subsystem
  Subsystem11 : Subsystem
  Subsystem12 : Subsystem
  Subsystem13 : Subsystem
  Subsystem14 : Subsystem
  Subsystem2 : Subsystem
  Subsystem3 : Subsystem
  Subsystem4 : Subsystem
  Subsystem5 : Subsystem
  Subsystem6 : Subsystem
  Subsystem7 : Subsystem
  Subsystem8 : Subsystem
  Subsystem9 : Subsystem
  BINP_TPMS_outputs : Outport  OutDataTypeStr=Bus: BINP_TPMS_outputs
  wires:
  Bus Selector/49 -> Data Type Conversion25/1  "<VHAL_S4ID_raw>"
  Bus Selector/48 -> Data Type Conversion24/1  "<VHAL_S3ID_raw>"
  Bus Selector/47 -> Data Type Conversion23/1  "<VHAL_S2ID_raw>"
  Bus Selector/46 -> Data Type Conversion22/1  "<VHAL_S1ID_raw>"
  Data Type Conversion25/1 -> Bus Creator/49  "VINP_S4ID_raw"
  Data Type Conversion24/1 -> Bus Creator/48  "VINP_S3ID_raw"
  Data Type Conversion23/1 -> Bus Creator/47  "VINP_S2ID_raw"
  Data Type Conversion22/1 -> Bus Creator/46  "VINP_S1ID_raw"
  Data Type Conversion21/1 -> Bus Creator/44  "VINP_FlashRRWheelTemp_C"
  Data Type Conversion20/1 -> Bus Creator/43  "VINP_FlashLRWheelTemp_C"
  Bus Selector/44 -> Data Type Conversion21/1  "<VHAL_FlashRRWheelTemp_C>"
  Bus Selector/43 -> Data Type Conversion20/1  "<VHAL_FlashLRWheelTemp_C>"
  Data Type Conversion55/1 -> Bus Creator/45  "VINP_FlashunlearnSfali_flg"
  Bus Selector/45 -> Data Type Conversion55/1  "<VHAL_FlashunlearnSfali_flg>"
  Data Type Conversion44/1 -> Bus Creator/42  "VINP_FlashRFWheelTemp_C"
  Bus Selector/42 -> Data Type Conversion44/1  "<VHAL_FlashRFWheelTemp_C>"
  Data Type Conversion43/1 -> Bus Creator/41  "VINP_FlashLFWheelTemp_C"
  Bus Selector/41 -> Data Type Conversion43/1  "<VHAL_FlashLFWheelTemp_C>"
  Data Type Conversion54/1 -> Bus Creator/40  "VINP_FlashRRWheelPress_raw8"
  Data Type Conversion42/1 -> Bus Creator/39  "VINP_FlashLRWheelPress_raw8"
  Bus Selector/40 -> Data Type Conversion54/1  "<VHAL_FlashRRWheelPress_raw8>"
  Bus Selector/39 -> Data Type Conversion42/1  "<VHAL_FlashLRWheelPress_raw8>"
  Data Type Conversion34/1 -> Bus Creator/38  "VINP_FlashRFWheelPress_raw8"
  Bus Selector/38 -> Data Type Conversion34/1  "<VHAL_FlashRFWheelPress_raw8>"
  Data Type Conversion56/1 -> Bus Creator/37  "VINP_FlashLFWheelPress_raw8"
  Bus Selector/37 -> Data Type Conversion56/1  "<VHAL_FlashLFWheelPress_raw8>"
  Data Type Conversion41/1 -> Bus Creator/36  "VINP_FlashRRP20_raw8"
  Bus Selector/36 -> Data Type Conversion41/1  "<VHAL_FlashRRP20_raw8>"
  Data Type Conversion39/1 -> Bus Creator/35  "VINP_FlashLRP20_raw8"
  Bus Selector/35 -> Data Type Conversion39/1  "<VHAL_FlashLRP20_raw8>"
  Data Type Conversion38/1 -> Bus Creator/34  "VINP_FlashRFP20_raw8"
  Bus Selector/34 -> Data Type Conversion38/1  "<VHAL_FlashRFP20_raw8>"
  Data Type Conversion40/1 -> Bus Creator/33  "VINP_FlashLFP20_raw8"
  Bus Selector/33 -> Data Type Conversion40/1  "<VHAL_FlashLFP20_raw8>"
  Data Type Conversion37/1 -> Bus Creator/32  "VINP_FlashRRPindi_enum"
  Bus Selector/32 -> Data Type Conversion37/1  "<VHAL_FlashRRPindi_enum>"
  Data Type Conversion35/1 -> Bus Creator/31  "VINP_FlashLRPindi_enum"
  Bus Selector/31 -> Data Type Conversion35/1  "<VHAL_FlashLRPindi_enum>"
  Data Type Conversion53/1 -> Bus Creator/30  "VINP_FlashRFPindi_enum"
  Bus Selector/30 -> Data Type Conversion53/1  "<VHAL_FlashRFPindi_enum>"
  Data Type Conversion32/1 -> Bus Creator/29  "VINP_FlashLFPindi_enum"
  Bus Selector/29 -> Data Type Conversion32/1  "<VHAL_FlashLFPindi_enum>"
  Data Type Conversion52/1 -> Bus Creator/28  "VINP_FlashRRWheelPSW_raw8"
  Bus Selector/28 -> Data Type Conversion52/1  "<VHAL_FlashRRWheelPSW_raw8>"
  Data Type Conversion50/1 -> Bus Creator/27  "VINP_FlashLRWheelPSW_raw8"
  Bus Selector/27 -> Data Type Conversion50/1  "<VHAL_FlashLRWheelPSW_raw8>"
  Data Type Conversion49/1 -> Bus Creator/26  "VINP_FlashRFWheelPSW_raw8"
  Bus Selector/26 -> Data Type Conversion49/1  "<VHAL_FlashRFWheelPSW_raw8>"
  Data Type Conversion51/1 -> Bus Creator/25  "VINP_FlashLFWheelPSW_raw8"
  Bus Selector/25 -> Data Type Conversion51/1  "<VHAL_FlashLFWheelPSW_raw8>"
  Data Type Conversion48/1 -> Bus Creator/24  "VINP_FlashRRSensorFail_flg"
  Bus Selector/24 -> Data Type Conversion48/1  "<VHAL_FlashRRSensorFail_flg>"
  Data Type Conversion47/1 -> Bus Creator/23  "VINP_FlashLRSensorFail_flg"
  Bus Selector/23 -> Data Type Conversion47/1  "<VHAL_FlashLRSensorFail_flg>"
  Data Type Conversion46/1 -> Bus Creator/22  "VINP_FlashRFSensorFail_flg"
  Bus Selector/22 -> Data Type Conversion46/1  "<VHAL_FlashRFSensorFail_flg>"
  Data Type Conversion45/1 -> Bus Creator/21  "VINP_FlashLFSensorFail_flg"
  Bus Selector/21 -> Data Type Conversion45/1  "<VHAL_FlashLFSensorFail_flg>"
  Data Type Conversion19/1 -> Bus Creator/20  "VINP_ChkRRID_raw"
  Data Type Conversion18/1 -> Bus Creator/19  "VINP_ChkLRID_raw"
  Data Type Conversion17/1 -> Bus Creator/18  "VINP_ChkRFID_raw"
  Data Type Conversion16/1 -> Bus Creator/17  "VINP_ChkLFID_raw"
  Data Type Conversion15/1 -> Bus Creator/16  "VINP_ChkStorge_flg"
  Bus Selector/20 -> Data Type Conversion19/1  "<VHAL_ChkRRID_raw>"
  Bus Selector/19 -> Data Type Conversion18/1  "<VHAL_ChkLRID_raw>"
  Bus Selector/18 -> Data Type Conversion17/1  "<VHAL_ChkRFID_raw>"
  Bus Selector/17 -> Data Type Conversion16/1  "<VHAL_ChkLFID_raw>"
  Bus Selector/16 -> Data Type Conversion15/1  "<VHAL_ChkStorge_flg>"
  Data Type Conversion14/1 -> Bus Creator/15  "VINP_RRID_raw"
  Data Type Conversion13/1 -> Bus Creator/14  "VINP_LRID_raw"
  Data Type Conversion12/1 -> Bus Creator/13  "VINP_RFID_raw"
  Data Type Conversion11/1 -> Bus Creator/12  "VINP_LFID_raw"
  Subsystem14/1(Out1) -> Data Type Conversion14/1
  Subsystem13/1(Out1) -> Data Type Conversion13/1
  Subsystem12/1(Out1) -> Data Type Conversion12/1
  Subsystem11/1(Out1) -> Data Type Conversion11/1
  Bus Selector/15 -> Subsystem14/1(In1)  "<VHAL_RRID_raw>"
  Bus Selector/14 -> Subsystem13/1(In1)  "<VHAL_LRID_raw>"
  Bus Selector/13 -> Subsystem12/1(In1)  "<VHAL_RFID_raw>"
  Bus Selector/12 -> Subsystem11/1(In1)  "<VHAL_LFID_raw>"
  Data Type Conversion10/1 -> Bus Creator/11  "VINP_TPMSStorge_flg"
  Subsystem10/1(Out1) -> Data Type Conversion10/1
  Bus Selector/11 -> Subsystem10/1(In1)  "<VHAL_TPMSStorge_flg>"
  Subsystem9/1(Out1) -> Data Type Conversion9/1
  Subsystem8/1(Out1) -> Data Type Conversion8/1
  Bus Selector/10 -> Subsystem9/1(In1)  "<VHAL_TPMSBattLow_flg>"
  Bus Selector/9 -> Subsystem8/1(In1)  "<VHAL_TPMSFAT_flg>"
  Data Type Conversion9/1 -> Bus Creator/10  "VINP_TPMSBattLow_flg"
  Data Type Conversion8/1 -> Bus Creator/9  "VINP_TPMSFAT_flg"
  Bus Creator/1 -> BINP_TPMS_outputs/1
  Data Type Conversion7/1 -> Bus Creator/8  "VINP_TPMSCRCCalc_crc"
  Data Type Conversion6/1 -> Bus Creator/7  "VINP_TPMSCRC_crc"
  Data Type Conversion5/1 -> Bus Creator/6  "VINP_TPMSPressureMi_raw"
  Data Type Conversion4/1 -> Bus Creator/5  "VINP_TPMSSta_enum"
  Data Type Conversion3/1 -> Bus Creator/4  "VINP_TPMSTemp_raw"
  Data Type Conversion2/1 -> Bus Creator/3  "VINP_TPMSPressure_raw"
  Data Type Conversion1/1 -> Bus Creator/2  "VINP_TPMSID_raw"
  Data Type Conversion/1 -> Bus Creator/1  "VINP_TPMSDataIn_flg"
  Subsystem7/1(Out1) -> Data Type Conversion7/1
  Subsystem6/1(Out1) -> Data Type Conversion6/1
  Subsystem5/1(Out1) -> Data Type Conversion5/1
  Subsystem4/1(Out1) -> Data Type Conversion4/1
  Subsystem3/1(Out1) -> Data Type Conversion3/1
  Subsystem2/1(Out1) -> Data Type Conversion2/1
  Subsystem1/1(Out1) -> Data Type Conversion1/1
  Subsystem/1(Out1) -> Data Type Conversion/1
  Bus Selector/8 -> Subsystem7/1(In1)  "<VHAL_TPMSCRCCalc_crc>"
  Bus Selector/7 -> Subsystem6/1(In1)  "<VHAL_TPMSCRC_crc>"
  Bus Selector/6 -> Subsystem5/1(In1)  "<VHAL_TPMSPressureMi_raw>"
  Bus Selector/5 -> Subsystem4/1(In1)  "<VHAL_TPMSSta_enum>"
  Bus Selector/4 -> Subsystem3/1(In1)  "<VHAL_TPMSTemp_raw>"
  Bus Selector/3 -> Subsystem2/1(In1)  "<VHAL_TPMSPressure_raw>"
  Bus Selector/2 -> Subsystem1/1(In1)  "<VHAL_TPMSID_raw>"
  Bus Selector/1 -> Subsystem/1(In1)  "<VHAL_TPMSDataIn_flg>"
  BHAL_TPMS_outputs/1 -> Bus Selector/1
  Bus Selector/50 -> Data Type Conversion26/1  "<VHAL_Prepresstemptrust_flg>"
  Data Type Conversion26/1 -> Bus Creator/50  "VINP_Prepresstemptrust_flg"

== system inp/INP/APM/Subsystem ==
  In1 : Inport
  Constant : Constant  Value=KINP_PASDRMR_cm_ovrdval
  Constant1 : Constant  Value=KINP_PASDRMR_cm_ovrdflg
  Switch : Switch  Criteria=u2 ~= 0
  Out1 : Outport
  wires:
  Switch/1 -> Out1/1
  In1/1 -> Switch/3
  Constant/1 -> Switch/1
  Constant1/1 -> Switch/2

== system inp/INP/APM/Subsystem1 ==
  In1 : Inport
  Constant : Constant  Value=KINP_PASDRML_cm_ovrdval
  Constant1 : Constant  Value=KINP_PASDRML_cm_ovrdflg
  Switch : Switch  Criteria=u2 ~= 0
  Out1 : Outport
  wires:
  Constant1/1 -> Switch/2
  Constant/1 -> Switch/1
  In1/1 -> Switch/3
  Switch/1 -> Out1/1

== system inp/INP/APM/Subsystem10 ==
  In1 : Inport
  Constant : Constant  Value=KINP_APSDFLR_cm_ovrdval
  Constant1 : Constant  Value=KINP_APSDFLR_cm_ovrdflg
  Switch : Switch  Criteria=u2 ~= 0
  Out1 : Outport
  wires:
  Switch/1 -> Out1/1
  In1/1 -> Switch/3
  Constant/1 -> Switch/1
  Constant1/1 -> Switch/2

== system inp/INP/APM/Subsystem11 ==
  In1 : Inport
  Constant : Constant  Value=KINP_APSDFLL_cm_ovrdval
  Constant1 : Constant  Value=KINP_APSDFLL_cm_ovrdflg
  Switch : Switch  Criteria=u2 ~= 0
  Out1 : Outport
  wires:
  Constant1/1 -> Switch/2
  Constant/1 -> Switch/1
  In1/1 -> Switch/3
  Switch/1 -> Out1/1

== system inp/INP/APM/Subsystem12 ==
  In1 : Inport
  Constant : Constant  Value=KINP_PASAFCL_enum_ovrdval
  Constant1 : Constant  Value=KINP_PASAFCL_enum_ovrdflg
  Switch : Switch  Criteria=u2 ~= 0
  Out1 : Outport
  wires:
  Switch/1 -> Out1/1
  In1/1 -> Switch/3
  Constant/1 -> Switch/1
  Constant1/1 -> Switch/2

== system inp/INP/APM/Subsystem13 ==
  In1 : Inport
  Constant : Constant  Value=KINP_PASARMR_enum_ovrdval
  Constant1 : Constant  Value=KINP_PASARMR_enum_ovrdflg
  Switch : Switch  Criteria=u2 ~= 0
  Out1 : Outport
  wires:
  Constant1/1 -> Switch/2
  Constant/1 -> Switch/1
  In1/1 -> Switch/3
  Switch/1 -> Out1/1

== system inp/INP/APM/Subsystem14 ==
  In1 : Inport
  Constant : Constant  Value=KINP_PASARML_enum_ovrdval
  Constant1 : Constant  Value=KINP_PASARML_enum_ovrdflg
  Switch : Switch  Criteria=u2 ~= 0
  Out1 : Outport
  wires:
  Switch/1 -> Out1/1
  In1/1 -> Switch/3
  Constant/1 -> Switch/1
  Constant1/1 -> Switch/2

== system inp/INP/APM/Subsystem15 ==
  In1 : Inport
  Constant : Constant  Value=KINP_PASARCR_enum_ovrdval
  Constant1 : Constant  Value=KINP_PASARCR_enum_ovrdflg
  Switch : Switch  Criteria=u2 ~= 0
  Out1 : Outport
  wires:
  Constant1/1 -> Switch/2
  Constant/1 -> Switch/1
  In1/1 -> Switch/3
  Switch/1 -> Out1/1

== system inp/INP/APM/Subsystem16 ==
  In1 : Inport
  Constant : Constant  Value=KINP_PASARCL_enum_ovrdval
  Constant1 : Constant  Value=KINP_PASARCL_enum_ovrdflg
  Switch : Switch  Criteria=u2 ~= 0
  Out1 : Outport
  wires:
  Switch/1 -> Out1/1
  In1/1 -> Switch/3
  Constant/1 -> Switch/1
  Constant1/1 -> Switch/2

== system inp/INP/APM/Subsystem17 ==
  In1 : Inport
  Constant : Constant  Value=KINP_PASAFMR_enum_ovrdval
  Constant1 : Constant  Value=KINP_PASAFMR_enum_ovrdflg
  Switch : Switch  Criteria=u2 ~= 0
  Out1 : Outport
  wires:
  Constant1/1 -> Switch/2
  Constant/1 -> Switch/1
  In1/1 -> Switch/3
  Switch/1 -> Out1/1

== system inp/INP/APM/Subsystem18 ==
  In1 : Inport
  Constant : Constant  Value=KINP_PASAFML_enum_ovrdval
  Constant1 : Constant  Value=KINP_PASAFML_enum_ovrdflg
  Switch : Switch  Criteria=u2 ~= 0
  Out1 : Outport
  wires:
  Switch/1 -> Out1/1
  In1/1 -> Switch/3
  Constant/1 -> Switch/1
  Constant1/1 -> Switch/2

== system inp/INP/APM/Subsystem19 ==
  In1 : Inport
  Constant : Constant  Value=KINP_PASAFCR_enum_ovrdval
  Constant1 : Constant  Value=KINP_PASAFCR_enum_ovrdflg
  Switch : Switch  Criteria=u2 ~= 0
  Out1 : Outport
  wires:
  Constant1/1 -> Switch/2
  Constant/1 -> Switch/1
  In1/1 -> Switch/3
  Switch/1 -> Out1/1

== system inp/INP/APM/Subsystem2 ==
  In1 : Inport
  Constant : Constant  Value=KINP_PASDRCR_cm_ovrdval
  Constant1 : Constant  Value=KINP_PASDRCR_cm_ovrdflg
  Switch : Switch  Criteria=u2 ~= 0
  Out1 : Outport
  wires:
  Constant1/1 -> Switch/2
  Constant/1 -> Switch/1
  In1/1 -> Switch/3
  Switch/1 -> Out1/1

== system inp/INP/APM/Subsystem20 ==
  In1 : Inport
  Constant : Constant  Value=KINP_USSStaRMR_flg_ovrdval
  Constant1 : Constant  Value=KINP_USSStaRMR_flg_ovrdflg
  Switch : Switch  Criteria=u2 ~= 0
  Out1 : Outport
  wires:
  Switch/1 -> Out1/1
  In1/1 -> Switch/3
  Constant/1 -> Switch/1
  Constant1/1 -> Switch/2

== system inp/INP/APM/Subsystem21 ==
  In1 : Inport
  Constant : Constant  Value=KINP_USSStaRML_flg_ovrdval
  Constant1 : Constant  Value=KINP_USSStaRML_flg_ovrdflg
  Switch : Switch  Criteria=u2 ~= 0
  Out1 : Outport
  wires:
  Constant1/1 -> Switch/2
  Constant/1 -> Switch/1
  In1/1 -> Switch/3
  Switch/1 -> Out1/1

== system inp/INP/APM/Subsystem22 ==
  In1 : Inport
  Constant : Constant  Value=KINP_USSStaRLR_flg_ovrdval
  Constant1 : Constant  Value=KINP_USSStaRLR_flg_ovrdflg
  Switch : Switch  Criteria=u2 ~= 0
  Out1 : Outport
  wires:
  Switch/1 -> Out1/1
  In1/1 -> Switch/3
  Constant/1 -> Switch/1
  Constant1/1 -> Switch/2

== system inp/INP/APM/Subsystem23 ==
  In1 : Inport
  Constant : Constant  Value=KINP_USSStaRLL_flg_ovrdval
  Constant1 : Constant  Value=KINP_USSStaRLL_flg_ovrdflg
  Switch : Switch  Criteria=u2 ~= 0
  Out1 : Outport
  wires:
  Constant1/1 -> Switch/2
  Constant/1 -> Switch/1
  In1/1 -> Switch/3
  Switch/1 -> Out1/1

== system inp/INP/APM/Subsystem24 ==
  In1 : Inport
  Constant : Constant  Value=KINP_USSStaRCR_flg_ovrdval
  Constant1 : Constant  Value=KINP_USSStaRCR_flg_ovrdflg
  Switch : Switch  Criteria=u2 ~= 0
  Out1 : Outport
  wires:
  Switch/1 -> Out1/1
  In1/1 -> Switch/3
  Constant/1 -> Switch/1
  Constant1/1 -> Switch/2

== system inp/INP/APM/Subsystem25 ==
  In1 : Inport
  Constant : Constant  Value=KINP_USSStaRCL_flg_ovrdval
  Constant1 : Constant  Value=KINP_USSStaRCL_flg_ovrdflg
  Switch : Switch  Criteria=u2 ~= 0
  Out1 : Outport
  wires:
  Constant1/1 -> Switch/2
  Constant/1 -> Switch/1
  In1/1 -> Switch/3
  Switch/1 -> Out1/1

== system inp/INP/APM/Subsystem26 ==
  In1 : Inport
  Constant : Constant  Value=KINP_USSStaFMR_flg_ovrdval
  Constant1 : Constant  Value=KINP_USSStaFMR_flg_ovrdflg
  Switch : Switch  Criteria=u2 ~= 0
  Out1 : Outport
  wires:
  Switch/1 -> Out1/1
  In1/1 -> Switch/3
  Constant/1 -> Switch/1
  Constant1/1 -> Switch/2

== system inp/INP/APM/Subsystem27 ==
  In1 : Inport
  Constant : Constant  Value=KINP_USSStaFML_flg_ovrdval
  Constant1 : Constant  Value=KINP_USSStaFML_flg_ovrdflg
  Switch : Switch  Criteria=u2 ~= 0
  Out1 : Outport
  wires:
  Constant1/1 -> Switch/2
  Constant/1 -> Switch/1
  In1/1 -> Switch/3
  Switch/1 -> Out1/1

== system inp/INP/APM/Subsystem28 ==
  In1 : Inport
  Constant : Constant  Value=KINP_USSStaFLR_flg_ovrdval
  Constant1 : Constant  Value=KINP_USSStaFLR_flg_ovrdflg
  Switch : Switch  Criteria=u2 ~= 0
  Out1 : Outport
  wires:
  Switch/1 -> Out1/1
  In1/1 -> Switch/3
  Constant/1 -> Switch/1
  Constant1/1 -> Switch/2

== system inp/INP/APM/Subsystem29 ==
  In1 : Inport
  Constant : Constant  Value=KINP_USSStaFLL_flg_ovrdval
  Constant1 : Constant  Value=KINP_USSStaFLL_flg_ovrdflg
  Switch : Switch  Criteria=u2 ~= 0
  Out1 : Outport
  wires:
  Constant1/1 -> Switch/2
  Constant/1 -> Switch/1
  In1/1 -> Switch/3
  Switch/1 -> Out1/1

== system inp/INP/APM/Subsystem3 ==
  In1 : Inport
  Constant : Constant  Value=KINP_PASDRCL_cm_ovrdval
  Constant1 : Constant  Value=KINP_PASDRCL_cm_ovrdflg
  Switch : Switch  Criteria=u2 ~= 0
  Out1 : Outport
  wires:
  Constant1/1 -> Switch/2
  Constant/1 -> Switch/1
  In1/1 -> Switch/3
  Switch/1 -> Out1/1

== system inp/INP/APM/Subsystem30 ==
  In1 : Inport
  Constant : Constant  Value=KINP_USSStaFCR_flg_ovrdval
  Constant1 : Constant  Value=KINP_USSStaFCR_flg_ovrdflg
  Switch : Switch  Criteria=u2 ~= 0
  Out1 : Outport
  wires:
  Switch/1 -> Out1/1
  In1/1 -> Switch/3
  Constant/1 -> Switch/1
  Constant1/1 -> Switch/2

== system inp/INP/APM/Subsystem31 ==
  In1 : Inport
  Constant : Constant  Value=KINP_USSStaFCL_flg_ovrdval
  Constant1 : Constant  Value=KINP_USSStaFCL_flg_ovrdflg
  Switch : Switch  Criteria=u2 ~= 0
  Out1 : Outport
  wires:
  Constant1/1 -> Switch/2
  Constant/1 -> Switch/1
  In1/1 -> Switch/3
  Switch/1 -> Out1/1

== system inp/INP/APM/Subsystem32 ==
  In1 : Inport
  Constant : Constant  Value=KINP_Chime_enum_ovrdval
  Constant1 : Constant  Value=KINP_Chime_enum_ovrdflg
  Switch : Switch  Criteria=u2 ~= 0
  Out1 : Outport
  wires:
  Switch/1 -> Out1/1
  In1/1 -> Switch/3
  Constant/1 -> Switch/1
  Constant1/1 -> Switch/2

== system inp/INP/APM/Subsystem33 ==
  In1 : Inport
  Constant : Constant  Value=KINP_SNSRLayout_enum_ovrdval
  Constant1 : Constant  Value=KINP_SNSRLayout_enum_ovrdflg
  Switch : Switch  Criteria=u2 ~= 0
  Out1 : Outport
  wires:
  Constant1/1 -> Switch/2
  Constant/1 -> Switch/1
  In1/1 -> Switch/3
  Switch/1 -> Out1/1

== system inp/INP/APM/Subsystem34 ==
  In1 : Inport
  Constant : Constant  Value=KINP_StaFSya_flg_ovrdval
  Constant1 : Constant  Value=KINP_StaFSya_flg_ovrdflg
  Switch : Switch  Criteria=u2 ~= 0
  Out1 : Outport
  wires:
  Switch/1 -> Out1/1
  In1/1 -> Switch/3
  Constant/1 -> Switch/1
  Constant1/1 -> Switch/2

== system inp/INP/APM/Subsystem35 ==
  In1 : Inport
  Constant : Constant  Value=KINP_ModOperation_enum_ovrdval
  Constant1 : Constant  Value=KINP_ModOperation_enum_ovrdflg
  Switch : Switch  Criteria=u2 ~= 0
  Out1 : Outport
  wires:
  Constant1/1 -> Switch/2
  Constant/1 -> Switch/1
  In1/1 -> Switch/3
  Switch/1 -> Out1/1

== system inp/INP/APM/Subsystem36 ==
  In1 : Inport
  Constant : Constant  Value=KINP_APSVMCReqA_flg_ovrflg
  Constant1 : Constant  Value=KINP_APSVMCReqA_flg_ovrdval
  Switch : Switch  Criteria=u2 ~= 0
  Out1 : Outport
  wires:
  Constant/1 -> Switch/2
  Constant1/1 -> Switch/1
  In1/1 -> Switch/3
  Switch/1 -> Out1/1

== system inp/INP/APM/Subsystem37 ==
  In1 : Inport
  Constant : Constant  Value=KINP_APSShiftPosnReq_enum_ovrflg
  Constant1 : Constant  Value=KINP_APSShiftPosnReq_enum_ovrdval
  Switch : Switch  Criteria=u2 ~= 0
  Out1 : Outport
  wires:
  Switch/1 -> Out1/1
  In1/1 -> Switch/3
  Constant1/1 -> Switch/1
  Constant/1 -> Switch/2
